simulink model "e_and_y_dot_2"  (R2018a)
settings: Solver=VariableStepAuto  StartTime=0.0  StopTime=time  RelTol=1e-3
values from neighbouring files (symbols this model uses):
  a11 = -2*(cf+cr)/m    (= -153.333333333)    [stab_anal.m]
  a12 = -1-2*(lf*cf-lr*cr)/m    (= 46.3333333333)    [stab_anal.m]
  a21 = -2*(lf*cf-lr*cr)/I    (= 28.4)    [stab_anal.m]
  a22 = -2*(lf*lf*cf+lr*lr*cr)/I    (= -176.12)    [stab_anal.m]
  b11 = 2*cf/m    (= 73.3333333333)    [stab_anal.m]
  b21 = 2*lf*cf/I    (= 48.4)    [stab_anal.m]
  G1 = 2.5    [stab_anal.m]
  G2 = -1.5    [stab_anal.m]
  G_d2g = 5    [stab_anal.m]
  I = 2500    [stab_anal.m]
  Kf = 55000    [stab_anal.m]
  Kr = 60000    [stab_anal.m]
  lf = 1.1    [stab_anal.m]
  lr = 1.6    [stab_anal.m]
  m = 1500    [stab_anal.m]
  n = 18.7    [stab_anal.m]
  sensitivity_e = 0.01    [stab_anal.m]
  sensitivity_y_dot = 0.01    [stab_anal.m]
  tau = 0.1    [stab_anal.m]
  V = 30/3.6    (= 8.33333333333)    [stab_anal.m]
settings Model: Creator=aoki-soya  LastModifiedBy=aoki-soya

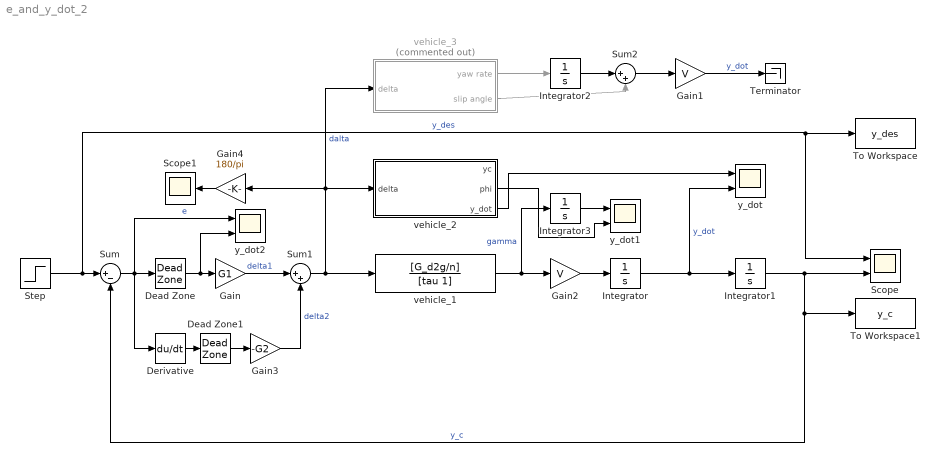
== system e_and_y_dot_2 ==
  Dead Zone : DeadZone  LowerValue=-sensitivity_e  UpperValue=sensitivity_e  SaturateOnIntegerOverflow=on
  Dead Zone1 : DeadZone  LowerValue=-sensitivity_y_dot  UpperValue=sensitivity_y_dot  SaturateOnIntegerOverflow=on
  Derivative : Derivative
  Gain : Gain  Gain=G1
  Gain1 : Gain  Gain=V
  Gain2 : Gain  Gain=V
  Gain3 : Gain  Gain=-G2
  Gain4 : Gain  Gain=180/pi
  Integrator{,1..3} (4 alike) : Integrator
  Scope : Scope  NumInputPorts=2
  Scope1 : Scope
  Step : Step  SampleTime=0
  Sum : Sum  Inputs=|+-
  Sum1 : Sum  Inputs=|++
  Sum2 : Sum  Inputs=|++
  Terminator : Terminator
  To Workspace : ToWorkspace  VariableName=y_des  SaveFormat=Timeseries  SampleTime=-1
  To Workspace1 : ToWorkspace  VariableName=y_c  SaveFormat=Timeseries  SampleTime=-1
  vehicle_1 : TransferFcn  Numerator=[G_d2g/n]  Denominator=[tau 1]
  vehicle_2 : Subsystem
  vehicle_3 : Subsystem  Commented=on
  y_dot : Scope  NumInputPorts=2
  y_dot1 : Scope  NumInputPorts=2
  y_dot2 : Scope  NumInputPorts=2
  wires:
  Step/1 -> Scope/1, To Workspace/1, Sum/1  "y_des"
  Sum/1 -> Derivative/1, y_dot2/1, Dead Zone/1  "e"
  Gain/1 -> Sum1/1  "delta1"
  Sum1/1 -> vehicle_2/1(delta), Gain4/1, vehicle_3/1(delta), vehicle_1/1  "dalta"
  vehicle_1/1 -> Integrator3/1, Gain2/1  "gamma"
  Gain2/1 -> Integrator/1
  Integrator1/1 -> Scope/2, To Workspace1/1, Sum/2  "y_c"
  Gain3/1 -> Sum1/2  "delta2"
  vehicle_3/1(yaw rate) -> Integrator2/1
  vehicle_3/2(slip angle) -> Sum2/2
  Integrator2/1 -> Sum2/1
  Sum2/1 -> Gain1/1
  Gain1/1 -> Terminator/1  "y_dot"
  Integrator/1 -> Integrator1/1, y_dot/2  "y_dot"
  vehicle_2/3(y_dot) -> y_dot/1
  Integrator3/1 -> y_dot1/1
  vehicle_2/2(phi) -> y_dot1/2
  Dead Zone1/1 -> Gain3/1
  Gain4/1 -> Scope1/1
  Dead Zone/1 -> y_dot2/2, Gain/1
  Derivative/1 -> Dead Zone1/1

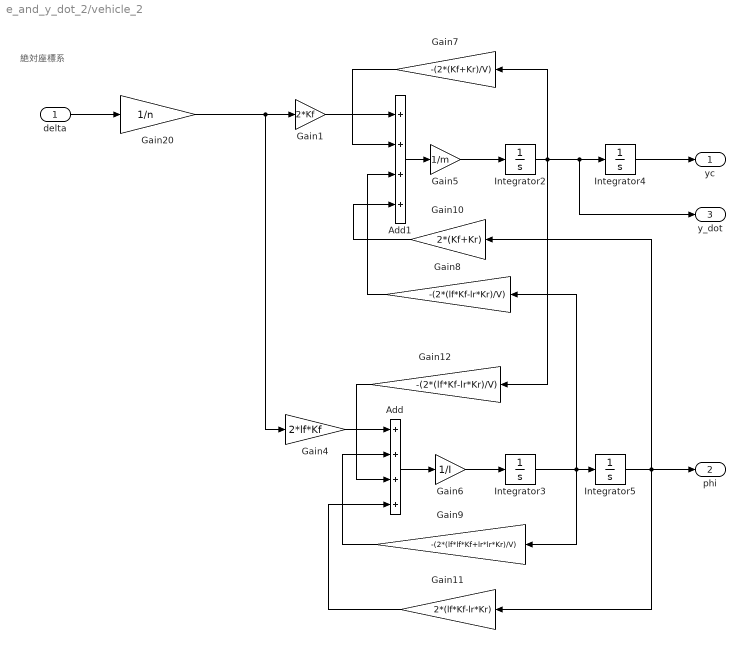
== system e_and_y_dot_2/vehicle_2 ==
  note: 絶対座標系
  delta : Inport
  Add : Sum  Inputs=++++
  Add1 : Sum  Inputs=++++
  Gain1 : Gain  Gain=2*Kf
  Gain10 : Gain  Gain=2*(Kf+Kr)
  Gain11 : Gain  Gain=2*(lf*Kf-lr*Kr)
  Gain12 : Gain  Gain=-(2*(lf*Kf-lr*Kr)/V)
  Gain20 : Gain  Gain=1/n
  Gain4 : Gain  Gain=2*lf*Kf
  Gain5 : Gain  Gain=1/m
  Gain6 : Gain  Gain=1/I
  Gain7 : Gain  Gain=-(2*(Kf+Kr)/V)
  Gain8 : Gain  Gain=-(2*(lf*Kf-lr*Kr)/V)
  Gain9 : Gain  Gain=-(2*(lf*lf*Kf+lr*lr*Kr)/V)
  Integrator{2..5} (4 alike) : Integrator
  yc : Outport
  phi : Outport  Port=2
  y_dot : Outport  Port=3
  wires:
  Gain6/1 -> Integrator3/1
  Integrator4/1 -> yc/1
  Add/1 -> Gain6/1
  Gain10/1 -> Add1/4
  Add1/1 -> Gain5/1
  Gain11/1 -> Add/4
  Gain8/1 -> Add1/3
  Gain5/1 -> Integrator2/1
  Gain1/1 -> Add1/1
  Gain9/1 -> Add/2
  Integrator3/1 -> Gain8/1, Integrator5/1, Gain9/1
  Integrator2/1 -> Gain7/1, Gain12/1, y_dot/1, Integrator4/1
  Gain4/1 -> Add/1
  Gain12/1 -> Add/3
  Integrator5/1 -> phi/1, Gain11/1, Gain10/1
  Gain7/1 -> Add1/2
  delta/1 -> Gain20/1
  Gain20/1 -> Gain4/1, Gain1/1

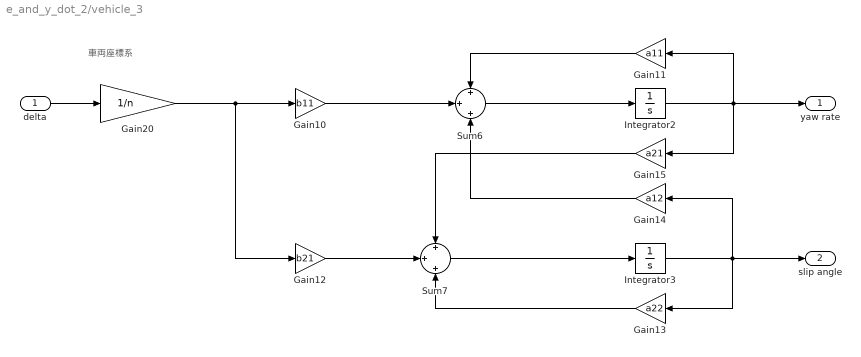
== system e_and_y_dot_2/vehicle_3 ==
  note: 車両座標系
  delta : Inport
  Gain10 : Gain  Gain=b11
  Gain11 : Gain  Gain=a11
  Gain12 : Gain  Gain=b21
  Gain13 : Gain  Gain=a22
  Gain14 : Gain  Gain=a12
  Gain15 : Gain  Gain=a21
  Gain20 : Gain  Gain=1/n
  Integrator2 : Integrator
  Integrator3 : Integrator
  Sum6 : Sum  Inputs=+|+|+
  Sum7 : Sum  Inputs=+|+|+
  yaw rate : Outport
  slip angle : Outport  Port=2
  wires:
  Gain10/1 -> Sum6/2
  Sum6/1 -> Integrator2/1
  Integrator2/1 -> Gain11/1, Gain15/1, yaw rate/1
  Gain11/1 -> Sum6/1
  Gain12/1 -> Sum7/2
  Sum7/1 -> Integrator3/1
  Integrator3/1 -> Gain14/1, Gain13/1, slip angle/1
  Gain13/1 -> Sum7/3
  Gain15/1 -> Sum7/1
  Gain14/1 -> Sum6/3
  Gain20/1 -> Gain12/1, Gain10/1
  delta/1 -> Gain20/1
